simulink model "propagatorSimple"  (R2023b)
settings: Solver=VariableStepAuto  StartTime=0.0  StopTime=tf  RelTol=1e-8  AbsTol=1e-8
undefined symbols (not defined in the file): area, burnOverride, initMass, juliandate, mDot, ref, thrust, thrustingThreshold, thrustingThresholdMn
libraries: vrlib x6, matrix_library x4, simulink x3
settings Model: SimulationMode=rapid-accelerator  Creator=miqui  LastModifiedBy=miqui

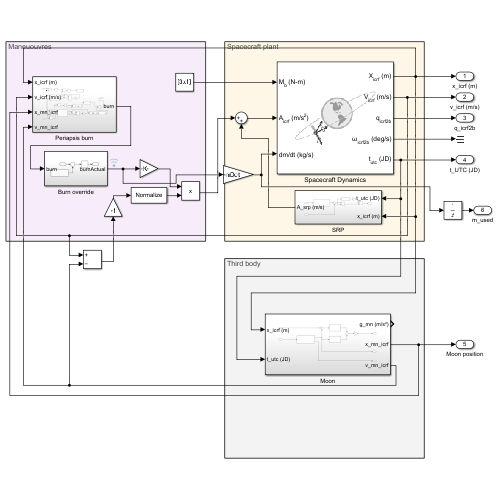
[thumbnail: Simulink's stored preview of the top-level diagram]
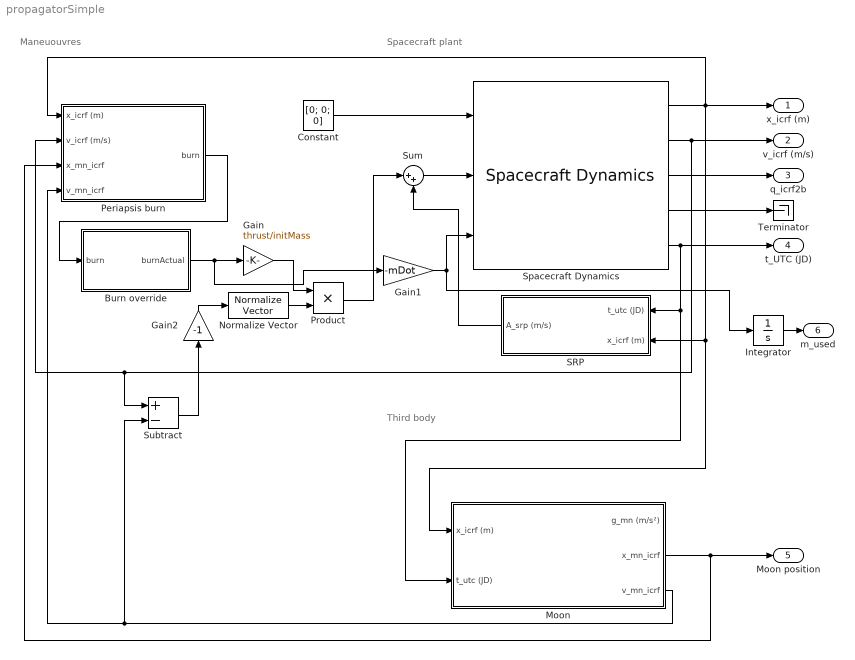
== system propagatorSimple ==
  note: Spacecraft plant
  note: Third body
  note: Maneuouvres
  Burn override : Subsystem
  Constant : Constant  Value=[0; 0; 0]
  Gain : Gain  Gain=thrust/initMass
  Gain1 : Gain  Gain=-mDot
  Gain2 : Gain  Gain=-1
  Integrator : Integrator
  Moon : Subsystem
  Normalize Vector : vrlib/Utilities/Normalize Vector  maxzero=0
  Periapsis burn : Subsystem
  Product : Product
  SRP : Subsystem
  Spacecraft Dynamics : SpacecraftDynamics  forcesIn=off  accelIn=on  startDate=startDate  massType=Simple variable  mass=initMass  emptyMass=endMass  fullMass=initMass  inertia=[1, 0, 0; 0, 1, 0; 0, 0, 1]*initMass  outputFuelStatus=off  semiMajorAxis=sma  eccentricity=ecc  inclination=inc  raan=RAAN  argPeriapsis=aop  trueAnomaly=true_an  useGravGrad=off  gravityModel=Oblate ellipsoid (J2)  useEOPs=off  useThirdBodyGravity=on  reflectivityCoeff=ref  srpArea=area
  Subtract : Sum  Inputs=+-
  Sum : Sum  Inputs=|++
  Terminator : Terminator
  x_icrf (m) : Outport
  v_icrf (m/s) : Outport  Port=2
  q_icrf2b : Outport  Port=3
  t_UTC (JD) : Outport  Port=4
  Moon position : Outport  Port=5
  m_used : Outport  Port=6
  wires:
  Spacecraft Dynamics/3 -> q_icrf2b/1
  Spacecraft Dynamics/2 -> Subtract/1, Periapsis burn/2(v_icrf (m/s)), v_icrf (m/s)/1
  Spacecraft Dynamics/5 -> SRP/1(t_utc (JD)), Moon/2(t_utc (JD)), t_UTC (JD)/1
  Moon/2(x_mn_icrf) -> Periapsis burn/3(x_mn_icrf), Moon position/1
  Spacecraft Dynamics/4 -> Terminator/1
  Spacecraft Dynamics/1 -> Periapsis burn/1(x_icrf (m)), SRP/2(x_icrf (m)), Moon/1(x_icrf (m)), x_icrf (m)/1
  Gain/1 -> Product/1
  Burn override/1(burnActual) -> Gain1/1, Gain/1
  Periapsis burn/1(burn) -> Burn override/1(burn)
  SRP/1(A_srp (m/s)) -> Sum/2
  Product/1 -> Sum/1
  Sum/1 -> Spacecraft Dynamics/2
  Constant/1 -> Spacecraft Dynamics/1
  Normalize Vector/1 -> Product/2
  Gain2/1 -> Normalize Vector/1
  Moon/3(v_mn_icrf) -> Subtract/2, Periapsis burn/4(v_mn_icrf)
  Gain1/1 -> Integrator/1, Spacecraft Dynamics/3
  Subtract/1 -> Gain2/1
  Integrator/1 -> m_used/1

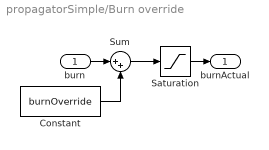
== system propagatorSimple/Burn override ==
  burn : Inport
  Constant : Constant  Value=burnOverride
  Saturation : Saturate  UpperLimit=1  LowerLimit=0
  Sum : Sum  Inputs=|++
  burnActual : Outport
  wires:
  Constant/1 -> Sum/2
  Saturation/1 -> burnActual/1
  burn/1 -> Sum/1
  Sum/1 -> Saturation/1

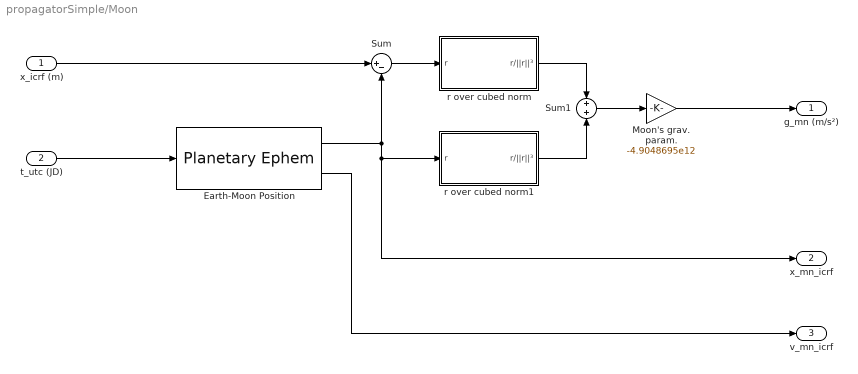
== system propagatorSimple/Moon ==
  x_icrf (m) : Inport
  t_utc (JD) : Inport  Port=2
  Earth-Moon Position : PlanetaryEphem  units=m,m/s  useDateRange=on  startDate=juliandate(2020,1,1)
  Moon's grav. param. : Gain  Gain=-4.9048695e12
  Sum : Sum  Inputs=|+-
  Sum1 : Sum
  r over cubed norm : Subsystem
  r over cubed norm1 : Subsystem
  g_mn (m/s²) : Outport
  x_mn_icrf : Outport  Port=2
  v_mn_icrf : Outport  Port=3
  wires:
  x_icrf (m)/1 -> Sum/1
  Earth-Moon Position/1 -> x_mn_icrf/1, r over cubed norm1/1(r), Sum/2
  Sum/1 -> r over cubed norm/1(r)
  Sum1/1 -> Moon's grav. param./1
  Moon's grav. param./1 -> g_mn (m/s²)/1
  r over cubed norm/1(r/||r||³) -> Sum1/1
  r over cubed norm1/1(r/||r||³) -> Sum1/2
  t_utc (JD)/1 -> Earth-Moon Position/1
  Earth-Moon Position/2 -> v_mn_icrf/1

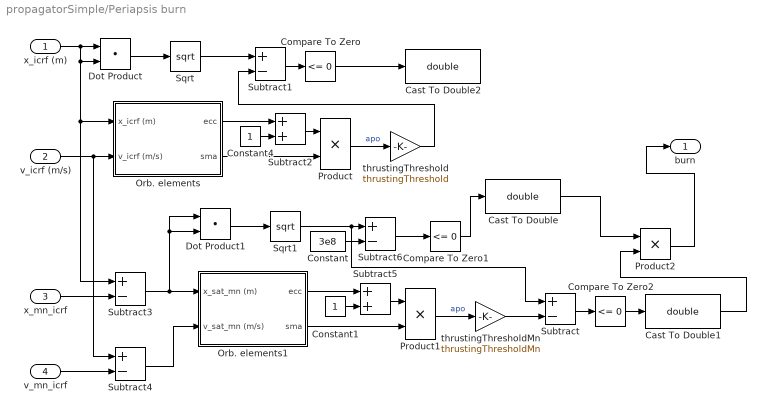
== system propagatorSimple/Periapsis burn ==
  x_icrf (m) : Inport
  v_icrf (m/s) : Inport  Port=2
  x_mn_icrf : Inport  Port=3
  v_mn_icrf : Inport  Port=4
  Cast To Double : DataTypeConversion  OutDataTypeStr=double  SaturateOnIntegerOverflow=off  RndMeth=Floor
  Cast To Double1 : DataTypeConversion  OutDataTypeStr=double  SaturateOnIntegerOverflow=off  RndMeth=Floor
  Cast To Double2 : DataTypeConversion  OutDataTypeStr=double  SaturateOnIntegerOverflow=off  RndMeth=Floor
  Compare To Zero : simulink/Logic and Bit Operations/Compare To Zero  relop=<=  OutDataTypeStr=boolean
  Compare To Zero1 : simulink/Logic and Bit Operations/Compare To Zero  relop=<=  OutDataTypeStr=boolean
  Compare To Zero2 : simulink/Logic and Bit Operations/Compare To Zero  relop=<=  OutDataTypeStr=boolean
  Constant : Constant  Value=3e8
  Constant1 : Constant
  Constant4 : Constant
  Dot Product : DotProduct  OutDataTypeStr=Inherit: Inherit via internal rule
  Dot Product1 : DotProduct  OutDataTypeStr=Inherit: Inherit via internal rule
  Orb. elements : Subsystem
  Orb. elements1 : Subsystem
  Product : Product
  Product1 : Product
  Product2 : Product
  Sqrt : Sqrt
  Sqrt1 : Sqrt
  Subtract{,1,3..4,6} (5 alike) : Sum  Inputs=+-
  Subtract2 : Sum
  Subtract5 : Sum
  thrustingThreshold : Gain  Gain=thrustingThreshold
  thrustingThresholdMn : Gain  Gain=thrustingThresholdMn
  burn : Outport
  wires:
  Dot Product/1 -> Sqrt/1
  Sqrt/1 -> Subtract1/1
  x_icrf (m)/1 -> Subtract3/1, Orb. elements/1(x_icrf (m)), Dot Product/2, Dot Product/1
  v_icrf (m/s)/1 -> Subtract4/1, Orb. elements/2(v_icrf (m/s))
  Subtract1/1 -> Compare To Zero/1
  Subtract2/1 -> Product/1
  Orb. elements/2(sma) -> Product/2
  thrustingThreshold/1 -> Subtract1/2
  Constant4/1 -> Subtract2/2
  Orb. elements/1(ecc) -> Subtract2/1
  x_mn_icrf/1 -> Subtract3/2
  v_mn_icrf/1 -> Subtract4/2
  Subtract4/1 -> Orb. elements1/2(v_sat_mn (m/s))
  Subtract3/1 -> Dot Product1/1, Dot Product1/2, Orb. elements1/1(x_sat_mn (m))
  Subtract5/1 -> Product1/1
  Orb. elements1/2(sma) -> Product1/2
  Constant1/1 -> Subtract5/2
  Orb. elements1/1(ecc) -> Subtract5/1
  Product/1 -> thrustingThreshold/1  "apo"
  Subtract6/1 -> Compare To Zero1/1
  Dot Product1/1 -> Sqrt1/1
  Sqrt1/1 -> Subtract/1, Subtract6/1
  Compare To Zero1/1 -> Cast To Double/1
  Constant/1 -> Subtract6/2
  Product1/1 -> thrustingThresholdMn/1  "apo"
  thrustingThresholdMn/1 -> Subtract/2
  Subtract/1 -> Compare To Zero2/1
  Compare To Zero2/1 -> Cast To Double1/1
  Cast To Double1/1 -> Product2/2
  Compare To Zero/1 -> Cast To Double2/1
  Cast To Double/1 -> Product2/1
  Product2/1 -> burn/1

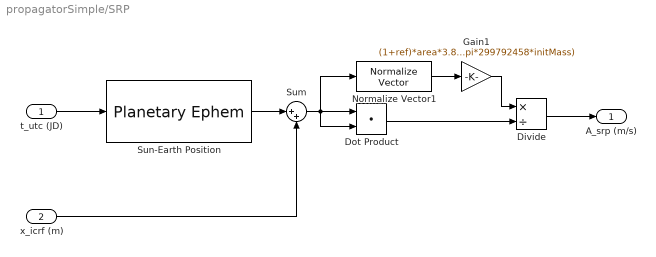
== system propagatorSimple/SRP ==
  t_utc (JD) : Inport
  x_icrf (m) : Inport  Port=2
  Divide : Product  Inputs=*/
  Dot Product : DotProduct  OutDataTypeStr=Inherit: Inherit via internal rule
  Gain1 : Gain  Gain=(1+ref)*area*3.852e26/(4*pi*299792458*initMass)
  Normalize Vector1 : vrlib/Utilities/Normalize Vector  maxzero=0
  Sum : Sum  Inputs=|++
  Sun-Earth Position : PlanetaryEphem  units=m,m/s  center=Sun  target=Earth  outputVelocity=off
  A_srp (m/s) : Outport
  wires:
  Normalize Vector1/1 -> Gain1/1
  Gain1/1 -> Divide/1
  Dot Product/1 -> Divide/2
  Divide/1 -> A_srp (m/s)/1
  t_utc (JD)/1 -> Sun-Earth Position/1
  Sun-Earth Position/1 -> Sum/1
  Sum/1 -> Dot Product/1, Normalize Vector1/1, Dot Product/2
  x_icrf (m)/1 -> Sum/2

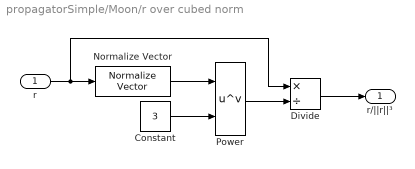
== system propagatorSimple/Moon/r over cubed norm ==
  r : Inport
  Constant : Constant  Value=3
  Divide : Product  Inputs=*/
  Normalize Vector : vrlib/Utilities/Normalize Vector  maxzero=0
  Power : Math  Operator=pow
  r/||r||³ : Outport
  wires:
  r/1 -> Divide/1, Normalize Vector/1
  Normalize Vector/1 -> Power/1
  Constant/1 -> Power/2
  Power/1 -> Divide/2
  Divide/1 -> r/||r||³/1

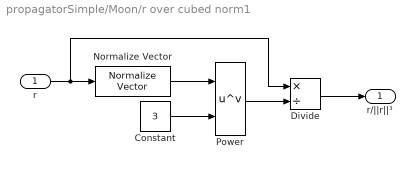
== system propagatorSimple/Moon/r over cubed norm1 ==
  r : Inport
  Constant : Constant  Value=3
  Divide : Product  Inputs=*/
  Normalize Vector : vrlib/Utilities/Normalize Vector  maxzero=0
  Power : Math  Operator=pow
  r/||r||³ : Outport
  wires:
  r/1 -> Divide/1, Normalize Vector/1
  Normalize Vector/1 -> Power/1
  Constant/1 -> Power/2
  Power/1 -> Divide/2
  Divide/1 -> r/||r||³/1

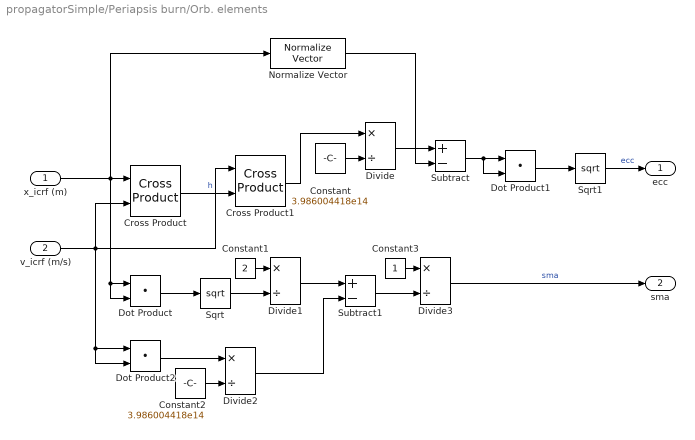
== system propagatorSimple/Periapsis burn/Orb. elements ==
  x_icrf (m) : Inport
  v_icrf (m/s) : Inport  Port=2
  Constant : Constant  Value=3.986004418e14
  Constant1 : Constant  Value=2
  Constant2 : Constant  Value=3.986004418e14
  Constant3 : Constant
  Cross Product : matrix_library/Cross Product
  Cross Product1 : matrix_library/Cross Product
  Divide{,1..3} (4 alike) : Product  Inputs=*/
  Dot Product : DotProduct  OutDataTypeStr=Inherit: Inherit via internal rule
  Dot Product1 : DotProduct  OutDataTypeStr=Inherit: Inherit via internal rule
  Dot Product2 : DotProduct  OutDataTypeStr=Inherit: Inherit via internal rule
  Normalize Vector : vrlib/Utilities/Normalize Vector  maxzero=0
  Sqrt : Sqrt
  Sqrt1 : Sqrt
  Subtract : Sum  Inputs=+-
  Subtract1 : Sum  Inputs=+-
  ecc : Outport
  sma : Outport  Port=2
  wires:
  x_icrf (m)/1 -> Normalize Vector/1, Dot Product/2, Dot Product/1, Cross Product/1
  v_icrf (m/s)/1 -> Dot Product2/2, Dot Product2/1, Cross Product1/1, Cross Product/2
  Cross Product/1 -> Cross Product1/2  "h"
  Constant/1 -> Divide/2
  Cross Product1/1 -> Divide/1
  Dot Product/1 -> Sqrt/1
  Sqrt/1 -> Divide1/2
  Divide/1 -> Subtract/1
  Normalize Vector/1 -> Subtract/2
  Dot Product1/1 -> Sqrt1/1
  Subtract/1 -> Dot Product1/2, Dot Product1/1
  Dot Product2/1 -> Divide2/1
  Constant1/1 -> Divide1/1
  Constant2/1 -> Divide2/2
  Divide1/1 -> Subtract1/1
  Divide2/1 -> Subtract1/2
  Subtract1/1 -> Divide3/2
  Constant3/1 -> Divide3/1
  Sqrt1/1 -> ecc/1  "ecc"
  Divide3/1 -> sma/1  "sma"

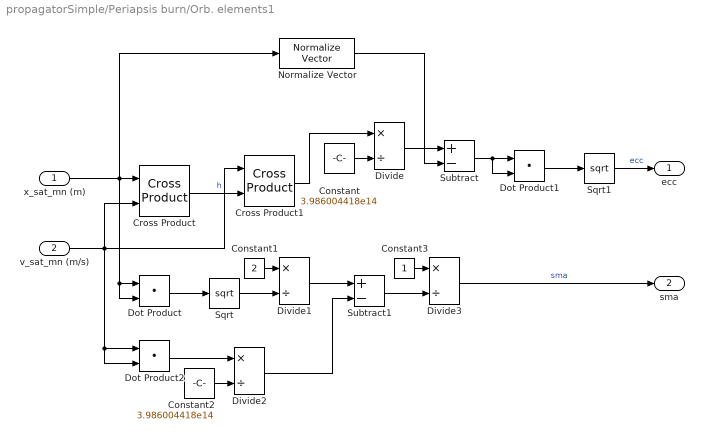
== system propagatorSimple/Periapsis burn/Orb. elements1 ==
  x_sat_mn (m) : Inport
  v_sat_mn (m/s) : Inport  Port=2
  Constant : Constant  Value=3.986004418e14
  Constant1 : Constant  Value=2
  Constant2 : Constant  Value=3.986004418e14
  Constant3 : Constant
  Cross Product : matrix_library/Cross Product
  Cross Product1 : matrix_library/Cross Product
  Divide{,1..3} (4 alike) : Product  Inputs=*/
  Dot Product : DotProduct  OutDataTypeStr=Inherit: Inherit via internal rule
  Dot Product1 : DotProduct  OutDataTypeStr=Inherit: Inherit via internal rule
  Dot Product2 : DotProduct  OutDataTypeStr=Inherit: Inherit via internal rule
  Normalize Vector : vrlib/Utilities/Normalize Vector  maxzero=0
  Sqrt : Sqrt
  Sqrt1 : Sqrt
  Subtract : Sum  Inputs=+-
  Subtract1 : Sum  Inputs=+-
  ecc : Outport
  sma : Outport  Port=2
  wires:
  x_sat_mn (m)/1 -> Normalize Vector/1, Dot Product/2, Dot Product/1, Cross Product/1
  v_sat_mn (m/s)/1 -> Dot Product2/2, Dot Product2/1, Cross Product1/1, Cross Product/2
  Cross Product/1 -> Cross Product1/2  "h"
  Constant/1 -> Divide/2
  Cross Product1/1 -> Divide/1
  Dot Product/1 -> Sqrt/1
  Sqrt/1 -> Divide1/2
  Divide/1 -> Subtract/1
  Normalize Vector/1 -> Subtract/2
  Dot Product1/1 -> Sqrt1/1
  Subtract/1 -> Dot Product1/2, Dot Product1/1
  Dot Product2/1 -> Divide2/1
  Constant1/1 -> Divide1/1
  Constant2/1 -> Divide2/2
  Divide1/1 -> Subtract1/1
  Divide2/1 -> Subtract1/2
  Subtract1/1 -> Divide3/2
  Constant3/1 -> Divide3/1
  Sqrt1/1 -> ecc/1  "ecc"
  Divide3/1 -> sma/1  "sma"
